simulink model "sfcndemo_dtype_param"  (Simulink 6.0)
settings: Solver=FixedStepDiscrete  StartTime=0.0  StopTime=10.0  RelTol=1e-3
settings Model: Creator=The MathWorks Inc.  LastModifiedBy=batserve  ExtModeAutoUpdateStatusClock=off
settings OptimizationCC: BlockReduction=off  BooleanDataType=off
settings DebuggingCC: CheckExecutionContextPreStartOutputMsg=on  CheckExecutionContextRuntimeOutputMsg=on  SolverPrmCheckMsg=none
settings HardwareCC: TargetUnknown=on

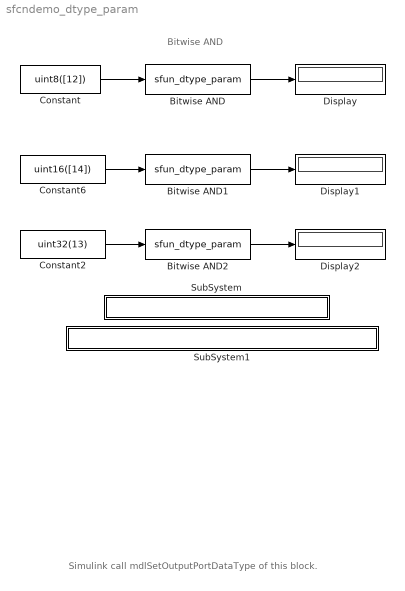
== system sfcndemo_dtype_param ==
  note: Simulink call mdlSetOutputPortDataType of this block.
  note: Bitwise AND
  Bitwise AND : S-Function  FunctionName=sfun_dtype_param  Parameters=uint8(11)
      settings: AttributesFormatString=%<Parameters>
  Bitwise AND1 : S-Function  FunctionName=sfun_dtype_param  Parameters=uint16(7)
      settings: AttributesFormatString=%<Parameters>
  Bitwise AND2 : S-Function  FunctionName=sfun_dtype_param  Parameters=uint32(6)
      settings: AttributesFormatString=%<Parameters>
  Constant : Constant  Value=uint8([12])
  Constant2 : Constant  Value=uint32(13)
  Constant6 : Constant  Value=uint16([14])
  Display : Display
  Display1 : Display
  Display2 : Display
  SubSystem : Subsystem  PropExecContextAcrossSSBoundary=on
      settings: OpenFcn=edit(fullfile(matlabroot,'simulink','src','sfun_dtype_param.c'))
      mask Display: disp('matlabroot\simulink\src\sfun_dtype_param.c');
  SubSystem1 : Subsystem  PropExecContextAcrossSSBoundary=on
      settings: OpenFcn=edit(fullfile(matlabroot,'toolbox','simulink','blocks','tlc_c','sfun_dtype_param.tlc'))
      mask Display: disp('matlabroot\toolbox\simulink\blocks\tlc_c\sfun_dtype_param.tlc');
  wires:
  Constant/1 -> Bitwise AND/1
  Bitwise AND/1 -> Display/1
  Constant6/1 -> Bitwise AND1/1
  Bitwise AND1/1 -> Display1/1
  Constant2/1 -> Bitwise AND2/1
  Bitwise AND2/1 -> Display2/1

== system sfcndemo_dtype_param/SubSystem ==

== system sfcndemo_dtype_param/SubSystem1 ==
